simulink model "TasksSimulink_OLD"  (R2016b)
settings: Solver=VariableStepAuto  StartTime=0.0  StopTime=36  RelTol=1e-3
values from neighbouring files (symbols this model uses):
  rollGrad = 5*(pi/180)    (= 0.0872664625997)    [UKF_start.m]
libraries: powerlib_meascontrol x2
settings Model: Creator=mitoa  LastModifiedBy=mitoa

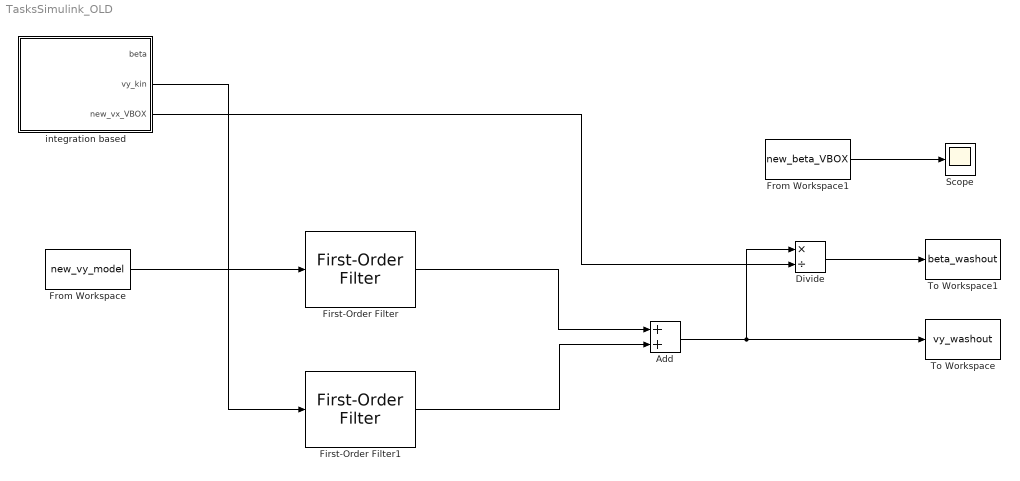
== system TasksSimulink_OLD ==
  Add : Sum
  Divide : Product  Inputs=*/
  First-Order Filter : powerlib_meascontrol/Filters/First-Order Filter  FilterType=Lowpass  Tc=T  Ts=0  Initialize=on  Vac_Init=[0, 0, 60]  Vdc_Init=0  PlotResponse=off  FreqRange="[0,  200,  1]"
  First-Order Filter1 : powerlib_meascontrol/Filters/First-Order Filter  FilterType=Highpass  Tc=T  Ts=0  Initialize=on  Vac_Init=[0, 0, 60]  Vdc_Init=0  PlotResponse=off  FreqRange="[0,  200,  1]"
  From Workspace : FromWorkspace  VariableName=new_vy_model  SampleTime=0
  From Workspace1 : FromWorkspace  VariableName=new_beta_VBOX  SampleTime=0
  Scope : Scope
  To Workspace : ToWorkspace  VariableName=vy_washout  SaveFormat=Timeseries  SampleTime=-1
  To Workspace1 : ToWorkspace  VariableName=beta_washout  SaveFormat=Timeseries  SampleTime=-1
  integration based : Subsystem
  wires:
  First-Order Filter/1 -> Add/1
  First-Order Filter1/1 -> Add/2
  From Workspace/1 -> First-Order Filter/1
  Add/1 -> Divide/1, To Workspace/1
  integration based/3(new_vx_VBOX) -> Divide/2
  Divide/1 -> To Workspace1/1
  integration based/2(vy_kin) -> First-Order Filter1/1
  From Workspace1/1 -> Scope/1

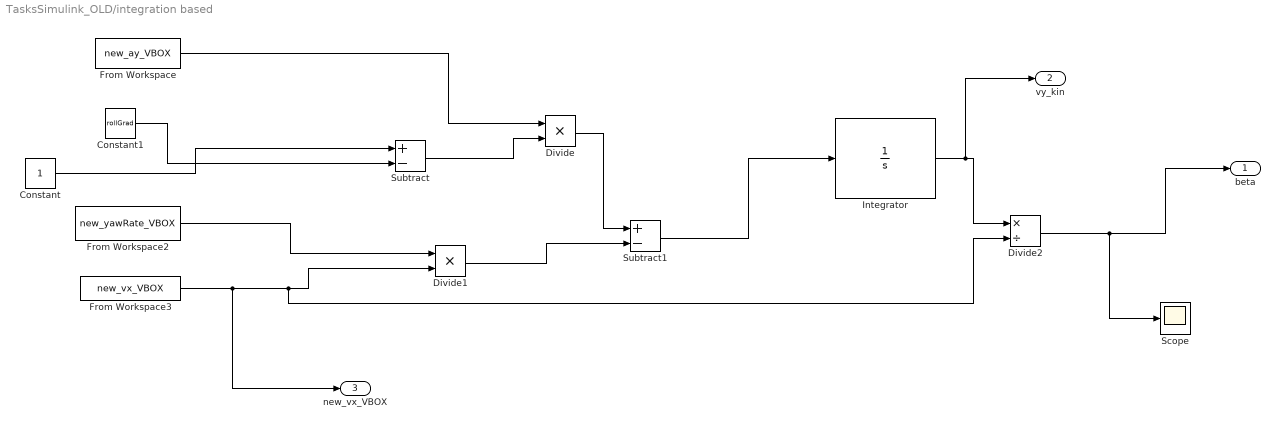
== system TasksSimulink_OLD/integration based ==
  Constant : Constant
  Constant1 : Constant  Value=rollGrad
  Divide : Product  Inputs=**
  Divide1 : Product  Inputs=**
  Divide2 : Product  Inputs=*/
  From Workspace : FromWorkspace  VariableName=new_ay_VBOX  SampleTime=0
  From Workspace2 : FromWorkspace  VariableName=new_yawRate_VBOX  SampleTime=0
  From Workspace3 : FromWorkspace  VariableName=new_vx_VBOX  SampleTime=0
  Integrator : Integrator
  Scope : Scope
  Subtract : Sum  Inputs=+-
  Subtract1 : Sum  Inputs=+-
  beta : Outport
  vy_kin : Outport  Port=2
  new_vx_VBOX : Outport  Port=3
  wires:
  Constant/1 -> Subtract/1
  Divide2/1 -> beta/1, Scope/1
  From Workspace/1 -> Divide/1
  Constant1/1 -> Subtract/2
  Subtract/1 -> Divide/2
  From Workspace3/1 -> new_vx_VBOX/1, Divide2/2, Divide1/2
  Subtract1/1 -> Integrator/1
  Divide/1 -> Subtract1/1
  Integrator/1 -> vy_kin/1, Divide2/1
  From Workspace2/1 -> Divide1/1
  Divide1/1 -> Subtract1/2
